simulink model "ACC_System"  (R2022a)
settings: Solver=FixedStepDiscrete  StartTime=0.0  StopTime=10.0  FixedStep=0.01  MaxStep=0.01  RelTol=1e-3
settings Model: DataDictionary=ACC_data_dictionary.sldd  EnableAccessToBaseWorkspace=off  Creator=jamesbond  LastModifiedBy=jamesbond
settings OptimizationCC: DefaultParameterBehavior=Inlined  EnhancedBackFolding=on  PassReuseOutputArgsAs=Individual arguments  ZeroExternalMemoryAtStartup=off  ZeroInternalMemoryAtStartup=off  OptimizeBlockOrder=speed  DifferentSizesBufferReuse=on  OptimizationCustomize=off  EfficientTunableParamExpr=on
settings DebuggingCC: ParameterTunabilityLossMsg=error
settings SFSimCC: MATLABDynamicMemAlloc=off
settings RTWCC: SystemTargetFile=ert.tlc  GenCodeOnly=on  TemplateMakefile=ert_default_tmf
settings CodeAppCC: ForceParamTrailComments=on  IgnoreCustomStorageClasses=off  OperatorAnnotations=on  SimulinkDataObjDesc=on  SFDataObjDesc=on  InsertBlockDesc=on
settings ERTTargetCC: TargetLangStandard=C99 (ISO)  GenerateSampleERTMain=on  InlinedParameterPlacement=NonHierarchical  ERTCustomFileTemplate=example_file_process.tlc
settings ConfigComp: CovMetricSettings=dcmrzoiwe

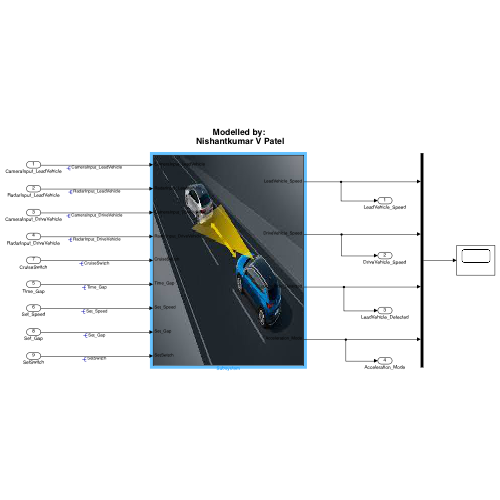
[thumbnail: Simulink's stored preview of the top-level diagram]
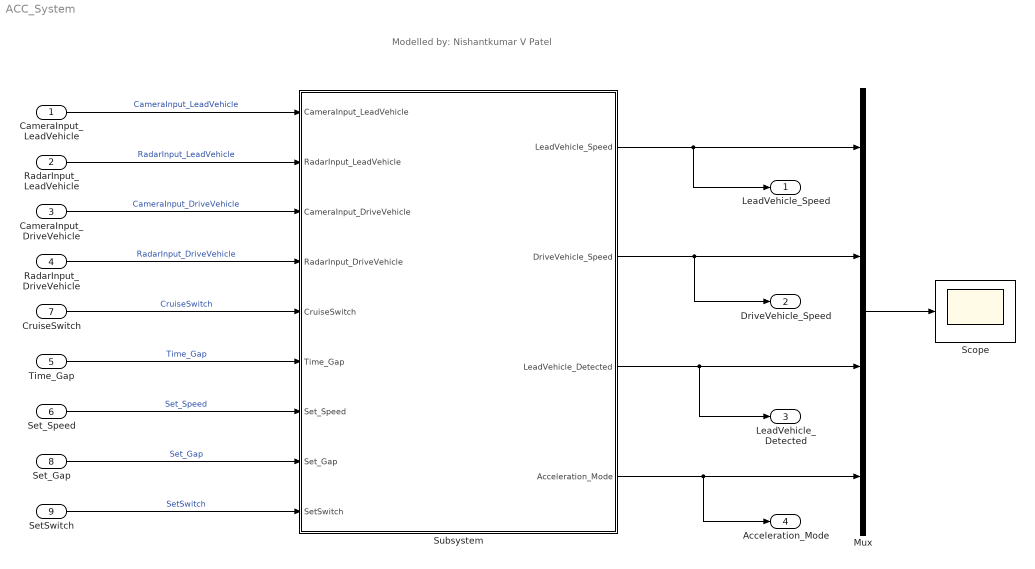
== system ACC_System ==
  note: Modelled by:
      | Nishantkumar V Patel
  CameraInput_LeadVehicle : Inport
  RadarInput_LeadVehicle : Inport  Port=2
  CameraInput_DriveVehicle : Inport  Port=3
  RadarInput_DriveVehicle : Inport  Port=4
  Time_Gap : Inport  Port=5
  Set_Speed : Inport  Port=6
  CruiseSwitch : Inport  Port=7
  Set_Gap : Inport  Port=8
  SetSwitch : Inport  Port=9
  Mux : Mux
  Scope : Scope
  Subsystem : Subsystem
      mask Display: image('$imagefile'); % Use "Edit Image" on toolstrip to change.
  LeadVehicle_Speed : Outport
  DriveVehicle_Speed : Outport  Port=2
  LeadVehicle_Detected : Outport  Port=3
  Acceleration_Mode : Outport  Port=4  OutDataTypeStr=uint8
  wires:
  CameraInput_LeadVehicle/1 -> Subsystem/1(CameraInput_LeadVehicle)  "CameraInput_LeadVehicle"
  RadarInput_LeadVehicle/1 -> Subsystem/2(RadarInput_LeadVehicle)  "RadarInput_LeadVehicle"
  CameraInput_DriveVehicle/1 -> Subsystem/3(CameraInput_DriveVehicle)  "CameraInput_DriveVehicle"
  RadarInput_DriveVehicle/1 -> Subsystem/4(RadarInput_DriveVehicle)  "RadarInput_DriveVehicle"
  Time_Gap/1 -> Subsystem/6(Time_Gap)  "Time_Gap"
  Set_Speed/1 -> Subsystem/7(Set_Speed)  "Set_Speed"
  Set_Gap/1 -> Subsystem/8(Set_Gap)  "Set_Gap"
  CruiseSwitch/1 -> Subsystem/5(CruiseSwitch)  "CruiseSwitch"
  SetSwitch/1 -> Subsystem/9(SetSwitch)  "SetSwitch"
  Subsystem/2(DriveVehicle_Speed) -> Mux/2, DriveVehicle_Speed/1
  Subsystem/1(LeadVehicle_Speed) -> LeadVehicle_Speed/1, Mux/1
  Subsystem/3(LeadVehicle_Detected) -> LeadVehicle_Detected/1, Mux/3
  Subsystem/4(Acceleration_Mode) -> Acceleration_Mode/1, Mux/4
  Mux/1 -> Scope/1

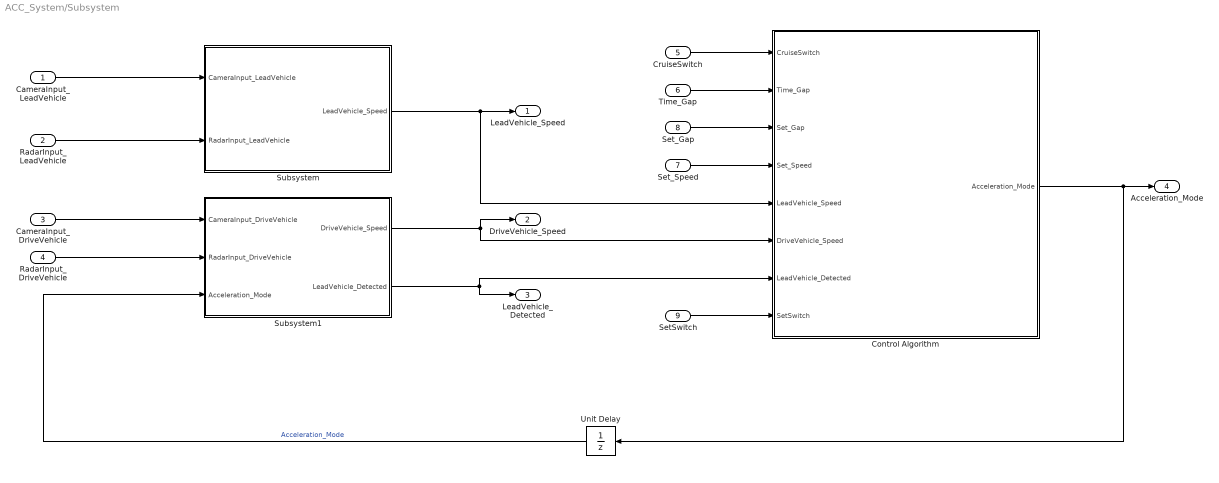
== system ACC_System/Subsystem ==
  CameraInput_LeadVehicle : Inport
  RadarInput_LeadVehicle : Inport  Port=2
  CameraInput_DriveVehicle : Inport  Port=3
  RadarInput_DriveVehicle : Inport  Port=4
  CruiseSwitch : Inport  Port=5
  Time_Gap : Inport  Port=6
  Set_Speed : Inport  Port=7
  Set_Gap : Inport  Port=8
  SetSwitch : Inport  Port=9
  Control Algorithm : Stateflow chart  TreatAsAtomicUnit=on
  Subsystem : Subsystem
  Subsystem1 : Subsystem
  Unit Delay : UnitDelay  SampleTime=-1  HasFrameUpgradeWarning=on
  LeadVehicle_Speed : Outport
  DriveVehicle_Speed : Outport  Port=2
  LeadVehicle_Detected : Outport  Port=3
  Acceleration_Mode : Outport  Port=4  OutDataTypeStr=uint8
  wires:
  CameraInput_LeadVehicle/1 -> Subsystem/1(CameraInput_LeadVehicle)
  RadarInput_LeadVehicle/1 -> Subsystem/2(RadarInput_LeadVehicle)
  CameraInput_DriveVehicle/1 -> Subsystem1/1(CameraInput_DriveVehicle)
  RadarInput_DriveVehicle/1 -> Subsystem1/2(RadarInput_DriveVehicle)
  Subsystem/1(LeadVehicle_Speed) -> LeadVehicle_Speed/1, Control Algorithm/5(LeadVehicle_Speed)
  Subsystem1/2(LeadVehicle_Detected) -> LeadVehicle_Detected/1, Control Algorithm/7(LeadVehicle_Detected)
  Subsystem1/1(DriveVehicle_Speed) -> DriveVehicle_Speed/1, Control Algorithm/6(DriveVehicle_Speed)
  CruiseSwitch/1 -> Control Algorithm/1(CruiseSwitch)
  Time_Gap/1 -> Control Algorithm/2(Time_Gap)
  Set_Gap/1 -> Control Algorithm/3(Set_Gap)
  Set_Speed/1 -> Control Algorithm/4(Set_Speed)
  Control Algorithm/1(Acceleration_Mode) -> Acceleration_Mode/1, Unit Delay/1
  Unit Delay/1 -> Subsystem1/3(Acceleration_Mode)  "Acceleration_Mode"
  SetSwitch/1 -> Control Algorithm/8(SetSwitch)

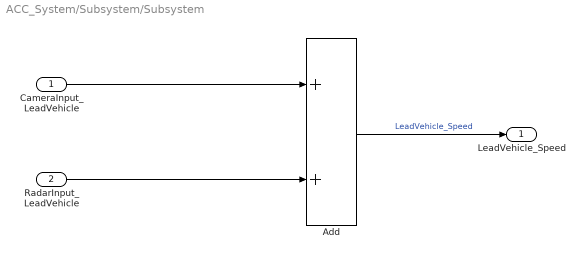
== system ACC_System/Subsystem/Subsystem ==
  CameraInput_LeadVehicle : Inport
  RadarInput_LeadVehicle : Inport  Port=2
  Add : Sum
  LeadVehicle_Speed : Outport
  wires:
  CameraInput_LeadVehicle/1 -> Add/1
  RadarInput_LeadVehicle/1 -> Add/2
  Add/1 -> LeadVehicle_Speed/1  "LeadVehicle_Speed"

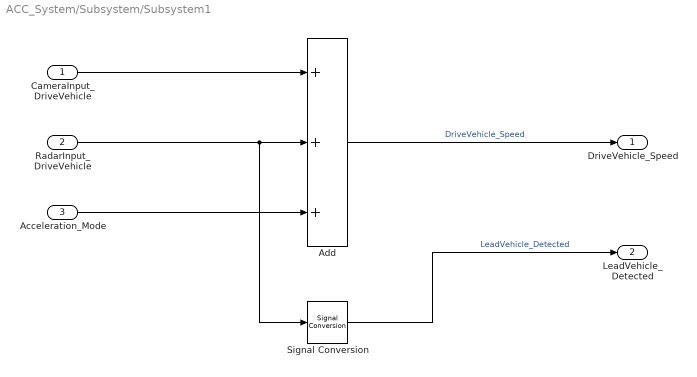
== system ACC_System/Subsystem/Subsystem1 ==
  CameraInput_DriveVehicle : Inport
  RadarInput_DriveVehicle : Inport  Port=2
  Acceleration_Mode : Inport  Port=3
  Add : Sum  Inputs=+++
  Signal Conversion : SignalConversion  OverrideOpt=off
  DriveVehicle_Speed : Outport
  LeadVehicle_Detected : Outport  Port=2
  wires:
  CameraInput_DriveVehicle/1 -> Add/1
  RadarInput_DriveVehicle/1 -> Signal Conversion/1, Add/2
  Acceleration_Mode/1 -> Add/3
  Signal Conversion/1 -> LeadVehicle_Detected/1  "LeadVehicle_Detected"
  Add/1 -> DriveVehicle_Speed/1  "DriveVehicle_Speed"

== stateflow chart ACC_System/Subsystem/Control Algorithm ==
  state ACC_OFF_Mode
    entry:
    Acceleration_Mode= 0;
  state ACC_STANDBY_Mode
    entry:
    Acceleration_Mode=1;
  state ACC_ON_Mode
    state LeadVehicle_Detected_Follow
      entry:
      Acceleration_Mode=2;
    state LeadVehicle_Detected_Resume
      entry:
      Acceleration_Mode=3;
    state LeadVehicle_Not_Detected_Resume
      entry:
      Acceleration_Mode=1;
    state LeadVehicle_Not_Detected
      entry:
      Acceleration_Mode=1;
    state LeadVehicle_Speed_lessthan_Set_Speed
      entry:
      Acceleration_Mode=4;
    state LeadVehicle_Speed_equal_Set_Speed
      entry:
      Acceleration_Mode=5;
    (default) -> LeadVehicle_Detected_Follow
    LeadVehicle_Detected_Resume -> LeadVehicle_Detected_Follow [order 3] : [(DriveVehicle_Speed == Set_Speed) && (LeadVehicle_Speed >= Set_Speed) && (Time_Gap >= Set_Gap)]
    LeadVehicle_Detected_Resume -> LeadVehicle_Not_Detected_Resume [order 1] : [LeadVehicle_Detected==0]
    LeadVehicle_Detected_Follow -> LeadVehicle_Not_Detected [order 1] : [ LeadVehicle_Detected == 0]
    LeadVehicle_Speed_equal_Set_Speed -> LeadVehicle_Not_Detected_Resume [order 3] : [(LeadVehicle_Detected == 0) || (DriveVehicle_Speed <= Set_Speed)]
    LeadVehicle_Speed_equal_Set_Speed -> LeadVehicle_Detected_Resume [order 2] : [(DriveVehicle_Speed < Set_Speed) && (LeadVehicle_Speed > DriveVehicle_Speed) || (Time_Gap >= Set_Gap)]
    LeadVehicle_Detected_Resume -> LeadVehicle_Speed_equal_Set_Speed [order 2] : [(DriveVehicle_Speed < Set_Speed) && (LeadVehicle_Speed > DriveVehicle_Speed) && (Time_Gap >= Set_Gap)]
    LeadVehicle_Not_Detected -> LeadVehicle_Detected_Follow [order 1] : [(LeadVehicle_Detected==1) && (DriveVehicle_Speed == Set_Speed) && (LeadVehicle_Speed >= Set_Speed) && (Time_Gap >= Set_Gap)]
    LeadVehicle_Detected_Follow -> LeadVehicle_Speed_lessthan_Set_Speed [order 2] : [(LeadVehicle_Detected == 1) && (LeadVehicle_Speed < Set_Speed) || (Time_Gap < Set_Gap)]
    LeadVehicle_Not_Detected -> LeadVehicle_Speed_lessthan_Set_Speed [order 2] : [(LeadVehicle_Detected == 1) && (LeadVehicle_Speed < Set_Speed) || (Time_Gap < Set_Gap)]
    LeadVehicle_Speed_lessthan_Set_Speed -> LeadVehicle_Not_Detected [order 2] : [(LeadVehicle_Detected == 0) && (DriveVehicle_Speed == Set_Speed)]
    LeadVehicle_Speed_lessthan_Set_Speed -> LeadVehicle_Speed_equal_Set_Speed [order 1] : [((LeadVehicle_Speed*1.25>=DriveVehicle_Speed) && (LeadVehicle_Speed * 0.75<=DriveVehicle_Speed)) && (DriveVehicle_Speed < Set_Speed) && ((Time_Gap<=1.25*Set_Gap) && (Time_Gap >=0.75*Set_Gap))]
    LeadVehicle_Speed_equal_Set_Speed -> LeadVehicle_Speed_lessthan_Set_Speed [order 1] : [(LeadVehicle_Speed<Set_Speed) && (LeadVehicle_Speed<DriveVehicle_Speed) || (Time_Gap == 0.75*Set_Gap)]
  (default) -> ACC_OFF_Mode
  ACC_STANDBY_Mode -> ACC_OFF_Mode [order 1] : [CruiseSwitch==0]
  ACC_OFF_Mode -> ACC_STANDBY_Mode : [CruiseSwitch==1]
  ACC_ON_Mode -> ACC_OFF_Mode [order 2] : [CruiseSwitch==0]
  ACC_STANDBY_Mode -> ACC_ON_Mode [order 2] : [SetSwitch==1]
  ACC_ON_Mode -> ACC_STANDBY_Mode [order 1] : [SetSwitch==0]
  data: CruiseSwitch input; Time_Gap input; Set_Gap input; Set_Speed input; Acceleration_Mode output; LeadVehicle_Speed input; DriveVehicle_Speed input; LeadVehicle_Detected input; SetSwitch input
